simulink model "QuadNHStepInput"  (R2017b)
settings: Solver=ode4  StartTime=0.0  StopTime=20  FixedStep=sim_step  RelTol=1e-3  EnableMultiTasking=on
values from neighbouring files (symbols this model uses):
  g = 9.81    [initNH.m]
  initlinvel = zeros(3,1)    [initNH.m]
  initpos = zeros(3,1)    [initNH.m]
  initRotMat = eye(3)    [initNH.m]
  initrotvel = zeros(3,1)    [initNH.m]
  J = diag([0.557, 0.557, 1.05]*10e-2)    [initNH.m]
  kd = 1.4*sqrt(4*kp)    [initNH.m]
  kd_z = kd    [initNH.m]
  KDP = 20    [initNH.m]
  KDR = 20    [initNH.m]
  KDY = 10    [initNH.m]
  ki = 1    [initNH.m]
  kp = 15    [initNH.m]
  KPP = 100    [initNH.m]
  KPR = 100    [initNH.m]
  m = 0.5    [initNH.m]
  max_pos_err_norm = 10    [initNH.m]
  max_tilt = 45/180*pi    (= 0.785398163397)    [initNH.m]
undefined symbols (not defined in the file or in its folder): setPos, setYaw
settings Model: Creator=Burak  LastModifiedBy=buyue
settings DataIOCC: LimitDataPoints=on  SaveFormat=Array
settings OptimizationCC: LifeSpan=inf
settings DebuggingCC: UnderspecifiedInitializationDetection=Classic  MergeDetectMultiDrivingBlocksExec=none  SolverPrmCheckMsg=warning  StateNameClashWarn=warning  SFUnexpectedBacktrackingDiag=warning  SFNoUnconditionalDefaultTransitionDiag=warning  SFExecutionAtInitializationDiag=none
settings HardwareCC: ProdBitPerPointer=32  ProdBitPerSizeT=32  ProdBitPerPtrDiffT=32  ProdLargestAtomicFloat=None  ProdIntDivRoundTo=Undefined  ProdEndianess=Unspecified  ProdWordSize=32  ProdHWDeviceType=32-bit Generic
settings ModelReferenceCC: PropagateSignalLabelsOutOfModel=off
settings CodeAppCC: StateflowObjectComments=on
settings GRTTargetCC: TargetLangStandard=C89/C90 (ANSI)  GeneratePreprocessorConditionals=Disable all
settings ConfigComp: CovMetricSettings=dw  CovHtmlReporting=on  CovSaveCumulativeToWorkspaceVar=on  CovSaveSingleToWorkspaceVar=on  CovExternalEMLEnable=off

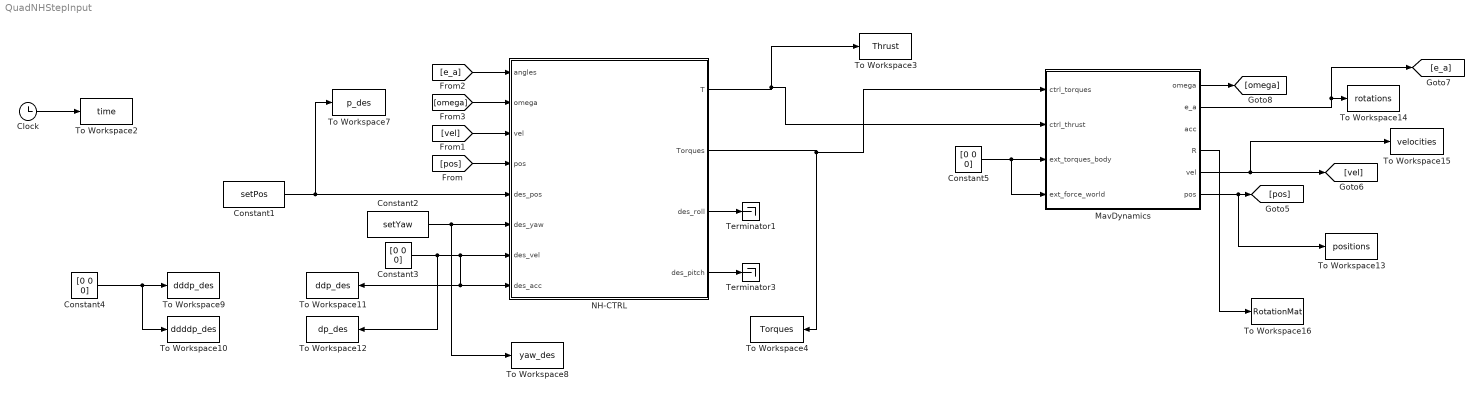
== system QuadNHStepInput ==
  Clock : Clock
  Constant1 : Constant  Value=setPos
  Constant2 : Constant  Value=setYaw
  Constant3 : Constant  Value=[0 0 0]
  Constant4 : Constant  Value=[0 0 0]
  Constant5 : Constant  Value=[0 0 0]
  MavDynamics : Subsystem
  NH-CTRL : Subsystem
  Terminator1 : Terminator
  Terminator3 : Terminator
  To Workspace10 : ToWorkspace  VariableName=ddddp_des  SampleTime=-1
  To Workspace11 : ToWorkspace  VariableName=ddp_des  SampleTime=-1
  To Workspace12 : ToWorkspace  VariableName=dp_des  SampleTime=-1
  To Workspace13 : ToWorkspace  VariableName=positions  SampleTime=-1
  To Workspace14 : ToWorkspace  VariableName=rotations  SampleTime=-1
  To Workspace15 : ToWorkspace  VariableName=velocities  SampleTime=-1
  To Workspace16 : ToWorkspace  VariableName=RotationMat  SampleTime=-1
  To Workspace2 : ToWorkspace  VariableName=time  SampleTime=-1
  To Workspace3 : ToWorkspace  VariableName=Thrust  SampleTime=-1
  To Workspace4 : ToWorkspace  VariableName=Torques  SampleTime=-1
  To Workspace7 : ToWorkspace  VariableName=p_des  SampleTime=-1
  To Workspace8 : ToWorkspace  VariableName=yaw_des  SampleTime=-1
  To Workspace9 : ToWorkspace  VariableName=dddp_des  SampleTime=-1
  wires:
  [e_a] -> NH-CTRL/1(angles)
  [omega] -> NH-CTRL/2(omega)
  [pos] -> NH-CTRL/4(pos)
  [vel] -> NH-CTRL/3(vel)
  NH-CTRL/3(des_roll) -> Terminator1/1
  NH-CTRL/4(des_pitch) -> Terminator3/1
  NH-CTRL/2(Torques) -> MavDynamics/1(ctrl_torques), To Workspace4/1
  NH-CTRL/1(T) -> MavDynamics/2(ctrl_thrust), To Workspace3/1
  Clock/1 -> To Workspace2/1
  Constant1/1 -> To Workspace7/1, NH-CTRL/5(des_pos)
  Constant2/1 -> To Workspace8/1, NH-CTRL/6(des_yaw)
  Constant3/1 -> To Workspace12/1, NH-CTRL/8(des_acc), To Workspace11/1, NH-CTRL/7(des_vel)
  Constant4/1 -> To Workspace10/1, To Workspace9/1
  MavDynamics/6(pos) -> To Workspace13/1, [pos]
  MavDynamics/2(e_a) -> [e_a], To Workspace14/1
  MavDynamics/1(omega) -> [omega]
  MavDynamics/4(R) -> To Workspace16/1
  MavDynamics/5(vel) -> To Workspace15/1, [vel]
  Constant5/1 -> MavDynamics/4(ext_force_world), MavDynamics/3(ext_torques_body)

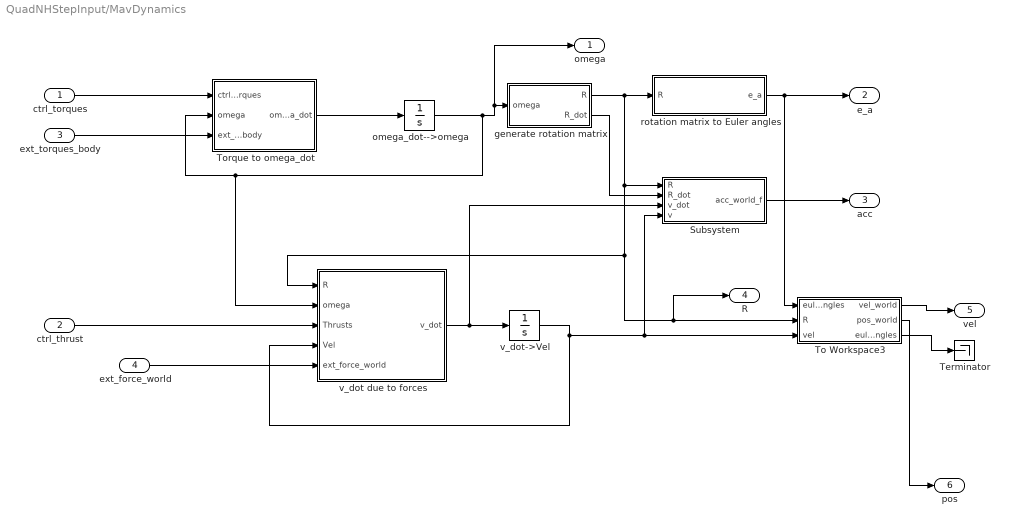
== system QuadNHStepInput/MavDynamics ==
  ctrl_torques : Inport
  ctrl_thrust : Inport  Port=2
  ext_torques_body : Inport  Port=3
  ext_force_world : Inport  Port=4
  Subsystem : Subsystem
  Terminator : Terminator
  To Workspace3 : Subsystem
  Torque to omega_dot : Subsystem
  generate rotation matrix : Subsystem
  omega_dot-->omega : Integrator  InitialCondition=initrotvel
  rotation matrix to Euler angles : MATLAB Function  TreatAsAtomicUnit=on
  v_dot due to forces : Subsystem
  v_dot->Vel : Integrator  InitialCondition=initlinvel
  omega : Outport
  e_a : Outport  Port=2
  acc : Outport  Port=3
  R : Outport  Port=4
  vel : Outport  Port=5
  pos : Outport  Port=6
  wires:
  To Workspace3/3("euler_angles ") -> Terminator/1
  v_dot due to forces/1(v_dot) -> Subsystem/3(v_dot), v_dot->Vel/1
  omega_dot-->omega/1 -> v_dot due to forces/2(omega), Torque to omega_dot/2(omega), omega/1, generate rotation matrix/1(omega)
  ext_force_world/1 -> v_dot due to forces/5(ext_force_world)
  To Workspace3/2(pos_world) -> pos/1
  Subsystem/1(acc_world_f) -> acc/1
  To Workspace3/1(vel_world) -> vel/1
  ctrl_thrust/1 -> v_dot due to forces/3(Thrusts)
  rotation matrix to Euler angles/1(e_a) -> e_a/1, To Workspace3/1(euler_angles)
  ext_torques_body/1 -> Torque to omega_dot/3(ext_torques_body)
  Torque to omega_dot/1(omega_dot) -> omega_dot-->omega/1
  generate rotation matrix/1(R) -> rotation matrix to Euler angles/1(R), R/1, To Workspace3/2(R), v_dot due to forces/1(R), Subsystem/1(R)
  v_dot->Vel/1 -> To Workspace3/3(vel), Subsystem/4(v), v_dot due to forces/4(Vel)
  generate rotation matrix/2(R_dot) -> Subsystem/2(R_dot)
  ctrl_torques/1 -> Torque to omega_dot/1(ctrl_orques)

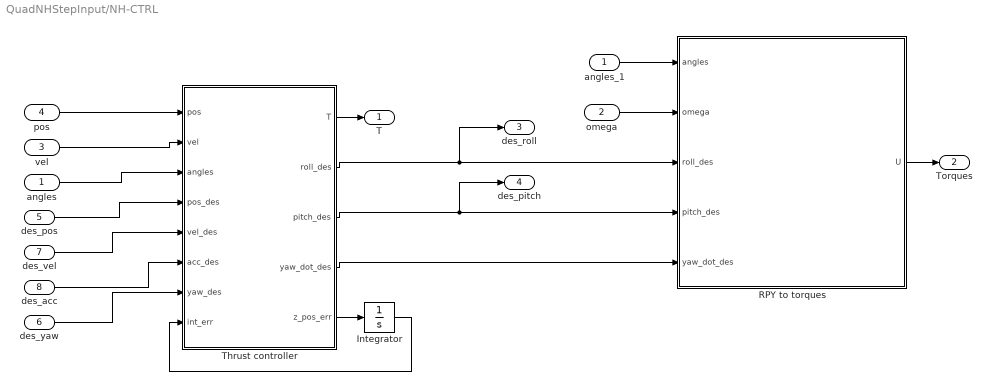
== system QuadNHStepInput/NH-CTRL ==
  angles : Inport
  omega : Inport  Port=2
  vel : Inport  Port=3
  pos : Inport  Port=4
  des_pos : Inport  Port=5
  des_yaw : Inport  Port=6
  des_vel : Inport  Port=7
  des_acc : Inport  Port=8
  Integrator : Integrator
  RPY to torques : MATLAB Function  TreatAsAtomicUnit=on
  Thrust controller : MATLAB Function  TreatAsAtomicUnit=on
  angles_1 : InportShadow
  T : Outport
  Torques : Outport  Port=2
  des_roll : Outport  Port=3
  des_pitch : Outport  Port=4
  wires:
  Integrator/1 -> Thrust controller/8(int_err)
  omega/1 -> RPY to torques/2(omega)
  vel/1 -> Thrust controller/2(vel)
  Thrust controller/3(pitch_des) -> des_pitch/1, RPY to torques/4(pitch_des)
  Thrust controller/4(yaw_dot_des) -> RPY to torques/5(yaw_dot_des)
  angles_1/1 -> RPY to torques/1(angles)
  des_acc/1 -> Thrust controller/6(acc_des)
  des_pos/1 -> Thrust controller/4(pos_des)
  des_yaw/1 -> Thrust controller/7(yaw_des)
  pos/1 -> Thrust controller/1(pos)
  Thrust controller/2(roll_des) -> des_roll/1, RPY to torques/3(roll_des)
  angles/1 -> Thrust controller/3(angles)
  Thrust controller/5(z_pos_err) -> Integrator/1
  des_vel/1 -> Thrust controller/5(vel_des)
  RPY to torques/1(U) -> Torques/1
  Thrust controller/1(T) -> T/1

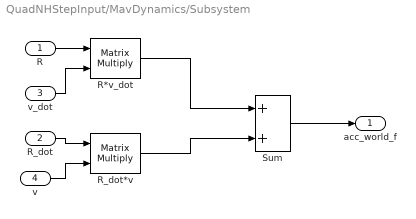
== system QuadNHStepInput/MavDynamics/Subsystem ==
  R : Inport
  R_dot : Inport  Port=2
  v_dot : Inport  Port=3
  v : Inport  Port=4
  R*v_dot : Product  Multiplication=Matrix(*)  RndMeth=Zero
  R_dot*v : Product  Multiplication=Matrix(*)  RndMeth=Zero
  Sum : Sum
  acc_world_f : Outport
  wires:
  Sum/1 -> acc_world_f/1
  R/1 -> R*v_dot/1
  v_dot/1 -> R*v_dot/2
  R_dot/1 -> R_dot*v/1
  v/1 -> R_dot*v/2
  R*v_dot/1 -> Sum/1
  R_dot*v/1 -> Sum/2

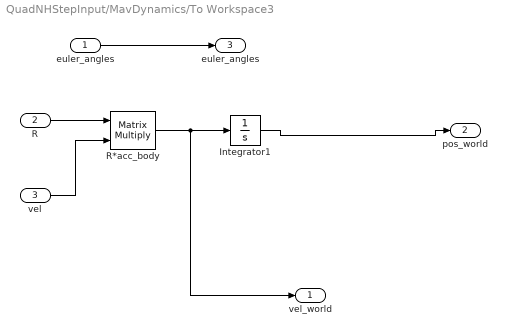
== system QuadNHStepInput/MavDynamics/To Workspace3 ==
  euler_angles : Inport
  R : Inport  Port=2
  vel : Inport  Port=3
  Integrator1 : Integrator  InitialCondition=initpos
  R*acc_body : Product  Multiplication=Matrix(*)  RndMeth=Zero
  vel_world : Outport
  pos_world : Outport  Port=2
  "euler_angles " : Outport  Port=3
  wires:
  R/1 -> R*acc_body/1
  vel/1 -> R*acc_body/2
  euler_angles/1 -> "euler_angles "/1
  R*acc_body/1 -> vel_world/1, Integrator1/1
  Integrator1/1 -> pos_world/1

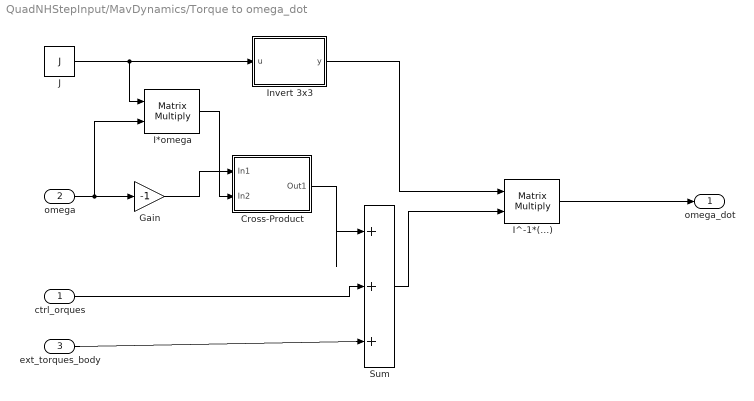
== system QuadNHStepInput/MavDynamics/Torque to omega_dot ==
  ctrl_orques : Inport
  omega : Inport  Port=2
  ext_torques_body : Inport  Port=3
  Cross-Product : Subsystem
  Gain : Gain  Gain=-1
  I*omega : Product  Multiplication=Matrix(*)  RndMeth=Zero
  I^-1*(...) : Product  Multiplication=Matrix(*)  RndMeth=Zero
  Invert 3x3 : MATLAB Function  TreatAsAtomicUnit=on
  J : Constant  Value=J
  Sum : Sum  Inputs=|+++
  omega_dot : Outport
  wires:
  omega/1 -> I*omega/2, Gain/1
  J/1 -> I*omega/1, Invert 3x3/1(u)
  I*omega/1 -> Cross-Product/2(In2)
  Invert 3x3/1(y) -> I^-1*(...)/1
  I^-1*(...)/1 -> omega_dot/1
  ctrl_orques/1 -> Sum/2
  Sum/1 -> I^-1*(...)/2
  Gain/1 -> Cross-Product/1(In1)
  Cross-Product/1(Out1) -> Sum/1
  ext_torques_body/1 -> Sum/3

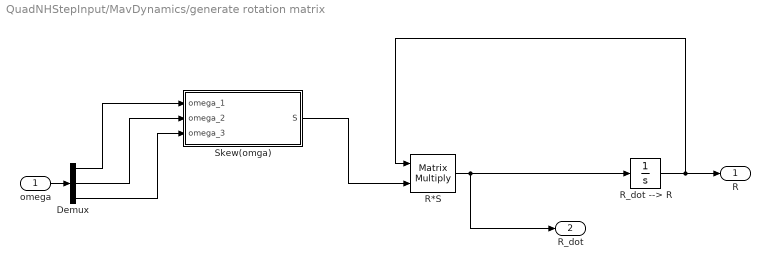
== system QuadNHStepInput/MavDynamics/generate rotation matrix ==
  omega : Inport
  Demux : Demux  Outputs=3
  R*S : Product  Multiplication=Matrix(*)  RndMeth=Zero
  R_dot --> R : Integrator  InitialCondition=initRotMat
  Skew(omga) : MATLAB Function  TreatAsAtomicUnit=on
  R : Outport
  R_dot : Outport  Port=2
  wires:
  R*S/1 -> R_dot --> R/1, R_dot/1
  R_dot --> R/1 -> R/1, R*S/1
  omega/1 -> Demux/1
  Demux/1 -> Skew(omga)/1(omega_1)
  Demux/2 -> Skew(omga)/2(omega_2)
  Demux/3 -> Skew(omga)/3(omega_3)
  Skew(omga)/1(S) -> R*S/2

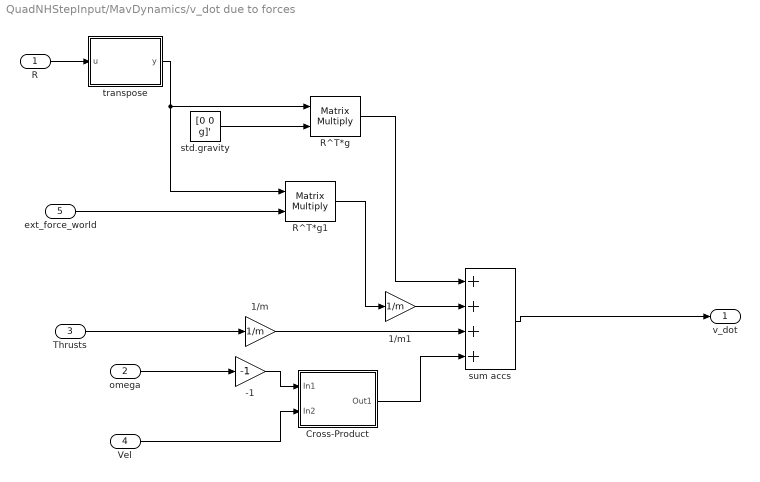
== system QuadNHStepInput/MavDynamics/v_dot due to forces ==
  R : Inport
  omega : Inport  Port=2
  Thrusts : Inport  Port=3
  Vel : Inport  Port=4
  ext_force_world : Inport  Port=5
  -1 : Gain  Gain=-1
  1/m : Gain  Gain=1/m
  1/m1 : Gain  Gain=1/m
  Cross-Product : Subsystem
  R^T*g : Product  Multiplication=Matrix(*)  RndMeth=Zero
  R^T*g1 : Product  Multiplication=Matrix(*)  RndMeth=Zero
  std.gravity : Constant  Value=[0 0 g]'
  sum accs : Sum  Inputs=++++
  transpose : MATLAB Function  TreatAsAtomicUnit=on
  v_dot : Outport
  wires:
  omega/1 -> -1/1
  Vel/1 -> Cross-Product/2(In2)
  R/1 -> transpose/1(u)
  transpose/1(y) -> R^T*g1/1, R^T*g/1
  std.gravity/1 -> R^T*g/2
  R^T*g/1 -> sum accs/1
  sum accs/1 -> v_dot/1
  Thrusts/1 -> 1/m/1
  -1/1 -> Cross-Product/1(In1)
  Cross-Product/1(Out1) -> sum accs/4
  1/m/1 -> sum accs/3
  ext_force_world/1 -> R^T*g1/2
  R^T*g1/1 -> 1/m1/1
  1/m1/1 -> sum accs/2

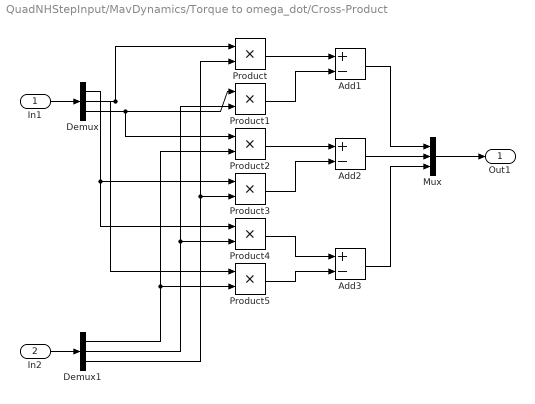
== system QuadNHStepInput/MavDynamics/Torque to omega_dot/Cross-Product ==
  In1 : Inport
  In2 : Inport  Port=2
  Add1 : Sum  Inputs=+-
  Add2 : Sum  Inputs=+-
  Add3 : Sum  Inputs=+-
  Demux : Demux  Outputs=3
  Demux1 : Demux  Outputs=3
  Mux : Mux  Inputs=3
  Product{,1..5} (6 alike) : Product  RndMeth=Zero
  Out1 : Outport
  wires:
  In1/1 -> Demux/1
  In2/1 -> Demux1/1
  Mux/1 -> Out1/1
  Add1/1 -> Mux/1
  Add2/1 -> Mux/2
  Add3/1 -> Mux/3
  Demux/2 -> Product/1, Product5/1
  Demux1/3 -> Product/2, Product3/2
  Demux/3 -> Product1/1, Product2/1
  Demux1/2 -> Product1/2, Product4/2
  Demux/1 -> Product3/1, Product4/1
  Demux1/1 -> Product2/2, Product5/2
  Product/1 -> Add1/1
  Product1/1 -> Add1/2
  Product2/1 -> Add2/1
  Product3/1 -> Add2/2
  Product4/1 -> Add3/1
  Product5/1 -> Add3/2

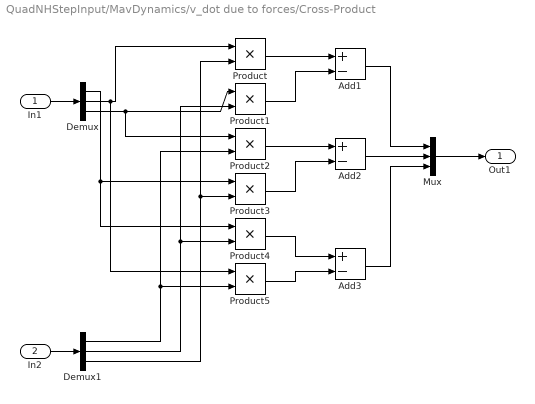
== system QuadNHStepInput/MavDynamics/v_dot due to forces/Cross-Product ==
  In1 : Inport
  In2 : Inport  Port=2
  Add1 : Sum  Inputs=+-
  Add2 : Sum  Inputs=+-
  Add3 : Sum  Inputs=+-
  Demux : Demux  Outputs=3
  Demux1 : Demux  Outputs=3
  Mux : Mux  Inputs=3
  Product{,1..5} (6 alike) : Product  RndMeth=Zero
  Out1 : Outport
  wires:
  In1/1 -> Demux/1
  In2/1 -> Demux1/1
  Mux/1 -> Out1/1
  Add1/1 -> Mux/1
  Add2/1 -> Mux/2
  Add3/1 -> Mux/3
  Demux/2 -> Product/1, Product5/1
  Demux1/3 -> Product/2, Product3/2
  Demux/3 -> Product1/1, Product2/1
  Demux1/2 -> Product1/2, Product4/2
  Demux/1 -> Product3/1, Product4/1
  Demux1/1 -> Product2/2, Product5/2
  Product/1 -> Add1/1
  Product1/1 -> Add1/2
  Product2/1 -> Add2/1
  Product3/1 -> Add2/2
  Product4/1 -> Add3/1
  Product5/1 -> Add3/2

== matlab function QuadNHStepInput/NH-CTRL/RPY to torques ==
  data: angles input; U output; omega input; roll_des input; pitch_des input; yaw_dot_des input; J parameter; KDR parameter; KPR parameter; KDP parameter; KPP parameter; KDY parameter
function U  = fcn(angles, omega, roll_des, pitch_des, yaw_dot_des, J, KDR, KPR, KDP, KPP, KDY)
% This block supports the Embedded MATLAB subset.
% See the help menu for details. 

% p = angles(2);
% r = angles(1);
% y=angles(3);
% 
% T = [1      tan(p)*sin(r) tan(p)*cos(r);
%     0       cos(r)  -sin(r);
%     0       sin(r)/cos(p)   cos(r)/cos(p)];
% 
% dot_ang = T*omega;
% dot_r=dot_ang(1);
% dot_p = dot_ang(2);
% 
% T_dot = [0  tan(p)*cos(r)*dot_r+(sin(r)+tan(p)^2*sin(r))*dot_p -tan(p)*sin(r)*dot_r+(cos(r)+tan(p)^2*cos(r))*dot_p;
%          0  -sin(r)*dot_r   -cos(r)*dot_r;
%          0  cos(r)/cos(p)*dot_r+sin(r)*sin(p)/cos(p)^2*dot_p    -sin(r)/cos(p)*dot_r+cos(r)*sin(p)/cos(p)^2*dot_p];
% 
% 
% k_d = 11;
% k_p = 30;
% ang_vel_des = [0 0 yaw_dot_des]';
% 
% 
% if(yaw_des - angles(3) > pi)
%     angles(3) = angles(3)+2*pi;
% elseif (yaw_des - angles(3) < -pi)
%     angles(3) = angles(3)-2*pi;
% end
% 
% ang_des = [roll_des pitch_des yaw_des]';
% U = I*inv(T)*(k_d*(ang_vel_des-dot_ang)+k_p*(ang_des - angles)-T_dot*omega)+cross(omega, I*omega);
% r_c = U(1);
% p_c = U(2);
% y_c = U(3);

U=[0;0;0];

r = angles(1);
p = angles(2);
y=angles(3);


T = [1      tan(p)*sin(r) tan(p)*cos(r);
    0       cos(r)  -sin(r);
    0       sin(r)/cos(p)   cos(r)/cos(p)];

dot_ang = T*omega;

dot_r= dot_ang(1);
dot_p = dot_ang(2);
dot_y = dot_ang(3);



% KDR = 20; 
% KPR = 100;
% 
% KDP = 20; 
% KPP = 100;
% 
% 
% KDY = 10;
% % KPY = 5;

Sw = [0 -omega(3) omega(2);                         % hat operation: R3->so3 (inverse of vee)
      omega(3) 0 -omega(1);
     -omega(2) omega(1) 0];

U=Sw*J*omega + J*inv(T)*([ KDR * (0 - dot_r) + KPR * (roll_des - r); KDP * (0 - dot_p) + KPP * (pitch_des - p) ; KDY * (yaw_dot_des - dot_y) ]);
% U=J*inv(T)*([ KDR * (0 - dot_r) + KPR * (roll_des - r); KDP * (0 - dot_p) + KPP * (pitch_des - p) ; KDY * (yaw_dot_des - dot_y) ]);


% U(1) = KDR * (0 - dot_r) + KPR * (roll_des - r);
% U(2) = KDP * (0 - dot_p) + KPP * (pitch_des - p);
% U(3) = KDY * (yaw_dot_des - dot_y);  %+ KPY * (yaw_des - y);
% 
% U=J*U;

== matlab function QuadNHStepInput/NH-CTRL/Thrust controller ==
  data: pos input; vel input; angles input; pos_des input; g parameter; m parameter; T output; roll_des output; pitch_des output; vel_des input; acc_des input; yaw_des input; yaw_dot_des output; kd parameter; kp parameter; ki parameter; max_tilt parameter; kd_z parameter; max_pos_err_norm parameter; int_err input; z_pos_err output
function [T, roll_des, pitch_des, yaw_dot_des,z_pos_err] = fcn(pos, vel, angles, pos_des, g, m, vel_des, acc_des,yaw_des, kd, kp, ki, max_tilt, kd_z, max_pos_err_norm,int_err)

r = angles(1);
p = angles(2);
y = angles(3);

pos_err = pos_des-pos;
T=zeros(3,1);

%hard saturation
% if norm(pos_err)>max_pos_err_norm
%     pos_err=pos_err/norm(pos_err)*max_pos_err_norm;
% end

%soft saturation
sat_norm = (2*max_pos_err_norm/pi) * atan( pi* norm(pos_err) / (2*max_pos_err_norm) );
if norm(pos_err) > 0.0001
    pos_err = pos_err/norm(pos_err) * sat_norm;
end

T=[0;0;m/(cos(r)*cos(p))*(-g+ acc_des(3) + kd_z*(vel_des(3) -vel(3)) + kp*(pos_err(3)) +ki*int_err )];


ddpx=kd*(vel_des(1) -vel(1)) + kp*(pos_err(1));
ddpy=kd*(vel_des(2) -vel(2)) + kp*(pos_err(2));

max_roll=sin(max_tilt);
max_pitch=sin(max_tilt);


ctrl_roll=m/T(3)*( -sin(y)*ddpx+cos(y)*ddpy);
ctrl_pitch= m/(T(3)*cos(r))*( cos(y)*ddpx+sin(y)*ddpy);


%hard saturation
% if abs(ctrl_roll)>max_roll
%     ctrl_roll=sign(ctrl_roll)*max_roll;
%     angle_sat=1;
% end
% 
% if abs(ctrl_pitch)>max_pitch
%     ctrl_pitch=sign(ctrl_pitch)*max_pitch;
%     angle_sat=1;
% end

%soft saturation
ctrl_roll = (2*max_roll/pi) * atan( pi* ctrl_roll / (2*max_roll) );

ctrl_pitch = (2*max_pitch/pi) * atan( pi* ctrl_pitch / (2*max_pitch) );

roll_des = -asin(ctrl_roll);

pitch_des = asin(ctrl_pitch);


% saturation
% if abs(roll_des) > max_tilt
%     
%     roll_des = sign(roll_des)*max_tilt;
%     
% end
% if abs(pitch_des) > max_tilt
%     
%     pitch_des = sign(pitch_des)*max_tilt;
%     
% end

z_pos_err = pos_err(3);

yaw_dot_des = kp*atan2(sin(yaw_des-y),cos(yaw_des-y));

== matlab function QuadNHStepInput/MavDynamics/Torque to omega_dot/Invert 3x3 ==
  data: u input; y output
function y = fcn(u)


y = NaN(3,3);
y(1,1) = u(3,3)*u(2,2)- u(2,3)*u(3,2);
y(1,2) = u(1,3)*u(3,2)- u(3,3)*u(1,2);
y(1,3) = u(1,2)*u(2,3)- u(2,2)*u(1,3);

y(2,1) = u(2,3)*u(3,1)- u(2,1)*u(3,3);
y(2,2) = u(1,1)*u(3,3)- u(3,1)*u(1,3);
y(2,3) = u(1,3)*u(2,1)- u(1,1)*u(2,3);

y(3,1) = u(2,1)*u(3,2)- u(2,2)*u(3,1);
y(3,2) = u(1,2)*u(3,1)- u(1,1)*u(3,2);
y(3,3) = u(1,1)*u(2,2)- u(1,2)*u(2,1);

y=1/det(u)*y;

== matlab function QuadNHStepInput/MavDynamics/generate rotation matrix/Skew(omga) ==
  data: omega_1 input; S output; omega_2 input; omega_3 input
function S = skew(omega_1, omega_2, omega_3)
% This block supports the Embedded MATLAB subset.
% See the help menu for details. 
S = [0 -omega_3 omega_2;
 omega_3 0 -omega_1;
 -omega_2 omega_1 0];

== matlab function QuadNHStepInput/MavDynamics/rotation matrix to Euler angles ==
  data: R input; e_a output
function e_a = eulerangles(R)
% This block supports an embeddable subset of the MATLAB language.
% See the help menu for details. 

e_a = zeros(3,1);

Roll = atan2(R(3,2),R(3,3));
Pitch = atan2(-R(3,1),sqrt(R(3,2)^2+R(3,3)^2));
Yaw = atan2(R(2,1),R(1,1));


e_a = [Roll; Pitch; Yaw];

== matlab function QuadNHStepInput/MavDynamics/v_dot due to forces/transpose ==
  data: u input; y output
function y = fcn(u)
% This block supports the Embedded MATLAB subset.
% See the help menu for details. 

y = u';
